simulink model "ship_template"  (R2021b)
settings: Solver=ode23t  StartTime=0.0  StopTime=60*2  MaxStep=0.1  RelTol=1e-3  AbsTol=1e-3
model workspace (MAT data in the model file):
  L = 1.2
  W = 1.2
undefined symbols (not defined in the file or in its folder): blue, blue0, blue1, blue2, centre, green, green0, green1, green2, left, Left, llx, lly, Mid, red, red0, red1, red2, right, Right, ulx, uly, X, Y, Z
libraries: sm_lib x278, nesl_utility x68, fl_lib x58, simulink x12, ee_lib x3, sdl_lib x3
(part 7 of 8)

== system ship_template/System/object scenario/9objs/contact models/object2ship/objectcontact ==
  Simscape Bus1 : SimscapeBus  HierarchyStrings=blue0;green0;red0;blue1;green1;red1;blue2;green2;red2
  Spatial Contact Force{1..6,9..11} (9 alike) : sm_lib/Forces and Torques/Spatial Contact Force  CoefficientOfDynamicFriction=0.3  CoefficientOfStaticFriction=0.5  SenseContactBaseRotation=off  SenseContactBaseTranslation=off  NormalDamping=b  NormalDampingUnits=N/(m/s)  SenseContactFollowerRotation=off  SenseContactFollowerTranslation=off  SenseContactSignal=off  NormalStiffness=k  NormalStiffnessUnits=N/m  FrictionalCriticalVelocity=1e-3  FrictionalCriticalVelocityUnits=m/s  ZeroCrossDetectContactStartAndEnd=off  FrictionType=SmoothStickSlip  SenseFrictionalForceMagnitude=off  SenseNormalForceMagnitude=off  NormalForceType=SmoothSpringDamper  SenseNormalVelocity=off  SenseSeparationDistance=off  SenseTangentialVelocity=off  SenseTangentialVelocityMagnitude=off  NormalTransitionRegionWidth=x  NormalTransitionRegionWidthUnits=m
  object : PMIOPort  Side=Left
  F : PMIOPort  Port=2  Side=Right
  connections:
  Spatial Contact Force11/RConn1 -- F/RConn1 -- Spatial Contact Force9/RConn1 -- Spatial Contact Force2/RConn1 -- Spatial Contact Force3/RConn1 -- Spatial Contact Force1/RConn1 -- Spatial Contact Force10/RConn1 -- Spatial Contact Force5/RConn1 -- Spatial Contact Force4/RConn1 -- Spatial Contact Force6/RConn1
  Spatial Contact Force10/LConn1 -- Simscape Bus1/LConn5
  Spatial Contact Force2/LConn1 -- Simscape Bus1/LConn3
  Spatial Contact Force3/LConn1 -- Simscape Bus1/LConn1
  Spatial Contact Force11/LConn1 -- Simscape Bus1/LConn6
  Spatial Contact Force1/LConn1 -- Simscape Bus1/LConn2
  Spatial Contact Force4/LConn1 -- Simscape Bus1/LConn8
  Spatial Contact Force9/LConn1 -- Simscape Bus1/LConn4
  Spatial Contact Force5/LConn1 -- Simscape Bus1/LConn9
  Spatial Contact Force6/LConn1 -- Simscape Bus1/LConn7
  Simscape Bus1/RConn1 -- object/RConn1

== system ship_template/System/object scenario/9objs/contact models/tank2collector/Subsystem ==
  Simscape Bus11 : SimscapeBus  HierarchyStrings=llx;ulx;lly;uly
  Spatial Contact Force{1,12,16..17} (4 alike) : sm_lib/Forces and Torques/Spatial Contact Force  CoefficientOfDynamicFriction=0.3  CoefficientOfStaticFriction=0.5  SenseContactBaseRotation=off  SenseContactBaseTranslation=off  NormalDamping=b  NormalDampingUnits=N/(m/s)  SenseContactFollowerRotation=off  SenseContactFollowerTranslation=off  SenseContactSignal=off  NormalStiffness=k  NormalStiffnessUnits=N/m  FrictionalCriticalVelocity=1e-3  FrictionalCriticalVelocityUnits=m/s  ZeroCrossDetectContactStartAndEnd=off  FrictionType=SmoothStickSlip  SenseFrictionalForceMagnitude=off  SenseNormalForceMagnitude=off  NormalForceType=SmoothSpringDamper  SenseNormalVelocity=off  SenseSeparationDistance=off  SenseTangentialVelocity=off  SenseTangentialVelocityMagnitude=off  NormalTransitionRegionWidth=x  NormalTransitionRegionWidthUnits=m
  tank wall : PMIOPort  Side=Left
  F : PMIOPort  Port=2  Side=Right
  connections:
  Simscape Bus11/LConn3 -- Spatial Contact Force16/LConn1
  Spatial Contact Force17/LConn1 -- Simscape Bus11/LConn1
  Spatial Contact Force16/RConn1 -- Spatial Contact Force1/RConn1 -- F/RConn1 -- Spatial Contact Force17/RConn1 -- Spatial Contact Force12/RConn1
  Simscape Bus11/LConn4 -- Spatial Contact Force1/LConn1
  tank wall/RConn1 -- Simscape Bus11/RConn1
  Simscape Bus11/LConn2 -- Spatial Contact Force12/LConn1

== system ship_template/System/object scenario/9objs/contact models/tank2collector/Subsystem1 ==
  Simscape Bus11 : SimscapeBus  HierarchyStrings=llx;ulx;lly;uly
  Spatial Contact Force{1,12,16..17} (4 alike) : sm_lib/Forces and Torques/Spatial Contact Force  CoefficientOfDynamicFriction=0.3  CoefficientOfStaticFriction=0.5  SenseContactBaseRotation=off  SenseContactBaseTranslation=off  NormalDamping=b  NormalDampingUnits=N/(m/s)  SenseContactFollowerRotation=off  SenseContactFollowerTranslation=off  SenseContactSignal=off  NormalStiffness=k  NormalStiffnessUnits=N/m  FrictionalCriticalVelocity=1e-3  FrictionalCriticalVelocityUnits=m/s  ZeroCrossDetectContactStartAndEnd=off  FrictionType=SmoothStickSlip  SenseFrictionalForceMagnitude=off  SenseNormalForceMagnitude=off  NormalForceType=SmoothSpringDamper  SenseNormalVelocity=off  SenseSeparationDistance=off  SenseTangentialVelocity=off  SenseTangentialVelocityMagnitude=off  NormalTransitionRegionWidth=x  NormalTransitionRegionWidthUnits=m
  tank wall : PMIOPort  Side=Left
  F : PMIOPort  Port=2  Side=Right
  connections:
  Simscape Bus11/LConn2 -- Spatial Contact Force12/LConn1
  tank wall/RConn1 -- Simscape Bus11/RConn1
  Simscape Bus11/LConn4 -- Spatial Contact Force1/LConn1
  F/RConn1 -- Spatial Contact Force12/RConn1 -- Spatial Contact Force17/RConn1 -- Spatial Contact Force16/RConn1 -- Spatial Contact Force1/RConn1
  Spatial Contact Force17/LConn1 -- Simscape Bus11/LConn1
  Simscape Bus11/LConn3 -- Spatial Contact Force16/LConn1

== system ship_template/System/object scenario/9objs/contact models/tank2collector/Subsystem2 ==
  Simscape Bus11 : SimscapeBus  HierarchyStrings=llx;ulx;lly;uly
  Spatial Contact Force{1,12,16..17} (4 alike) : sm_lib/Forces and Torques/Spatial Contact Force  CoefficientOfDynamicFriction=0.3  CoefficientOfStaticFriction=0.5  SenseContactBaseRotation=off  SenseContactBaseTranslation=off  NormalDamping=b  NormalDampingUnits=N/(m/s)  SenseContactFollowerRotation=off  SenseContactFollowerTranslation=off  SenseContactSignal=off  NormalStiffness=k  NormalStiffnessUnits=N/m  FrictionalCriticalVelocity=1e-3  FrictionalCriticalVelocityUnits=m/s  ZeroCrossDetectContactStartAndEnd=off  FrictionType=SmoothStickSlip  SenseFrictionalForceMagnitude=off  SenseNormalForceMagnitude=off  NormalForceType=SmoothSpringDamper  SenseNormalVelocity=off  SenseSeparationDistance=off  SenseTangentialVelocity=off  SenseTangentialVelocityMagnitude=off  NormalTransitionRegionWidth=x  NormalTransitionRegionWidthUnits=m
  tank wall : PMIOPort  Side=Left
  F : PMIOPort  Port=2  Side=Right
  connections:
  Simscape Bus11/LConn3 -- Spatial Contact Force16/LConn1
  Spatial Contact Force17/LConn1 -- Simscape Bus11/LConn1
  Spatial Contact Force1/RConn1 -- Spatial Contact Force16/RConn1 -- Spatial Contact Force17/RConn1 -- Spatial Contact Force12/RConn1 -- F/RConn1
  Simscape Bus11/LConn4 -- Spatial Contact Force1/LConn1
  tank wall/RConn1 -- Simscape Bus11/RConn1
  Simscape Bus11/LConn2 -- Spatial Contact Force12/LConn1

== system ship_template/System/object scenario/9objs/objects/object location/checkCollected ==
  xy : Inport
  Compare To Constant : simulink/Logic and Bit Operations/Compare To Constant  relop=<=  const=homeRadius  OutDataTypeStr=boolean
  Constant : Constant  Value=[Xhome, Yhome]
  Sqrt : Sqrt  SaturateOnIntegerOverflow=on
  Square : Math  Operator=square  SaturateOnIntegerOverflow=on
  Sum : Sum  Inputs=|-+
  Sum of Elements : Sum  Inputs=+
  collectFlag : Outport
  wires:
  Sum of Elements/1 -> Sqrt/1
  Sqrt/1 -> Compare To Constant/1  "dist"
  xy/1 -> Sum/1
  Square/1 -> Sum of Elements/1
  Compare To Constant/1 -> collectFlag/1  "collected"
  Constant/1 -> Sum/2
  Sum/1 -> Square/1

== system ship_template/System/object scenario/9objs/objects/object location/checkCollected1 ==
  xy : Inport
  Compare To Constant : simulink/Logic and Bit Operations/Compare To Constant  relop=<=  const=homeRadius  OutDataTypeStr=boolean
  Constant : Constant  Value=[Xhome, Yhome]
  Sqrt : Sqrt  SaturateOnIntegerOverflow=on
  Square : Math  Operator=square  SaturateOnIntegerOverflow=on
  Sum : Sum  Inputs=|-+
  Sum of Elements : Sum  Inputs=+
  collectFlag : Outport
  wires:
  Sum/1 -> Square/1
  Constant/1 -> Sum/2
  Compare To Constant/1 -> collectFlag/1  "collected"
  Square/1 -> Sum of Elements/1
  xy/1 -> Sum/1
  Sqrt/1 -> Compare To Constant/1  "dist"
  Sum of Elements/1 -> Sqrt/1

== system ship_template/System/object scenario/9objs/objects/object location/checkCollected2 ==
  xy : Inport
  Compare To Constant : simulink/Logic and Bit Operations/Compare To Constant  relop=<=  const=homeRadius  OutDataTypeStr=boolean
  Constant : Constant  Value=[Xhome, Yhome]
  Sqrt : Sqrt  SaturateOnIntegerOverflow=on
  Square : Math  Operator=square  SaturateOnIntegerOverflow=on
  Sum : Sum  Inputs=|-+
  Sum of Elements : Sum  Inputs=+
  collectFlag : Outport
  wires:
  Sum of Elements/1 -> Sqrt/1
  Sqrt/1 -> Compare To Constant/1  "dist"
  xy/1 -> Sum/1
  Square/1 -> Sum of Elements/1
  Compare To Constant/1 -> collectFlag/1  "collected"
  Constant/1 -> Sum/2
  Sum/1 -> Square/1

== system ship_template/System/object scenario/9objs/objects/object location/checkCollected3 ==
  xy : Inport
  Compare To Constant : simulink/Logic and Bit Operations/Compare To Constant  relop=<=  const=homeRadius  OutDataTypeStr=boolean
  Constant : Constant  Value=[Xhome, Yhome]
  Sqrt : Sqrt  SaturateOnIntegerOverflow=on
  Square : Math  Operator=square  SaturateOnIntegerOverflow=on
  Sum : Sum  Inputs=|-+
  Sum of Elements : Sum  Inputs=+
  collectFlag : Outport
  wires:
  Sum/1 -> Square/1
  Constant/1 -> Sum/2
  Compare To Constant/1 -> collectFlag/1  "collected"
  Square/1 -> Sum of Elements/1
  xy/1 -> Sum/1
  Sqrt/1 -> Compare To Constant/1  "dist"
  Sum of Elements/1 -> Sqrt/1

== system ship_template/System/object scenario/9objs/objects/object location/checkCollected4 ==
  xy : Inport
  Compare To Constant : simulink/Logic and Bit Operations/Compare To Constant  relop=<=  const=homeRadius  OutDataTypeStr=boolean
  Constant : Constant  Value=[Xhome, Yhome]
  Sqrt : Sqrt  SaturateOnIntegerOverflow=on
  Square : Math  Operator=square  SaturateOnIntegerOverflow=on
  Sum : Sum  Inputs=|-+
  Sum of Elements : Sum  Inputs=+
  collectFlag : Outport
  wires:
  Sum of Elements/1 -> Sqrt/1
  Sqrt/1 -> Compare To Constant/1  "dist"
  xy/1 -> Sum/1
  Square/1 -> Sum of Elements/1
  Compare To Constant/1 -> collectFlag/1  "collected"
  Constant/1 -> Sum/2
  Sum/1 -> Square/1

== system ship_template/System/object scenario/9objs/objects/object location/checkCollected5 ==
  xy : Inport
  Compare To Constant : simulink/Logic and Bit Operations/Compare To Constant  relop=<=  const=homeRadius  OutDataTypeStr=boolean
  Constant : Constant  Value=[Xhome, Yhome]
  Sqrt : Sqrt  SaturateOnIntegerOverflow=on
  Square : Math  Operator=square  SaturateOnIntegerOverflow=on
  Sum : Sum  Inputs=|-+
  Sum of Elements : Sum  Inputs=+
  collectFlag : Outport
  wires:
  Sum/1 -> Square/1
  Constant/1 -> Sum/2
  Compare To Constant/1 -> collectFlag/1  "collected"
  Square/1 -> Sum of Elements/1
  xy/1 -> Sum/1
  Sqrt/1 -> Compare To Constant/1  "dist"
  Sum of Elements/1 -> Sqrt/1

== system ship_template/System/object scenario/9objs/objects/object location/checkCollected6 ==
  xy : Inport
  Compare To Constant : simulink/Logic and Bit Operations/Compare To Constant  relop=<=  const=homeRadius  OutDataTypeStr=boolean
  Constant : Constant  Value=[Xhome, Yhome]
  Sqrt : Sqrt  SaturateOnIntegerOverflow=on
  Square : Math  Operator=square  SaturateOnIntegerOverflow=on
  Sum : Sum  Inputs=|-+
  Sum of Elements : Sum  Inputs=+
  collectFlag : Outport
  wires:
  Sum of Elements/1 -> Sqrt/1
  Sqrt/1 -> Compare To Constant/1  "dist"
  xy/1 -> Sum/1
  Square/1 -> Sum of Elements/1
  Compare To Constant/1 -> collectFlag/1  "collected"
  Constant/1 -> Sum/2
  Sum/1 -> Square/1

== system ship_template/System/object scenario/9objs/objects/object location/checkCollected7 ==
  xy : Inport
  Compare To Constant : simulink/Logic and Bit Operations/Compare To Constant  relop=<=  const=homeRadius  OutDataTypeStr=boolean
  Constant : Constant  Value=[Xhome, Yhome]
  Sqrt : Sqrt  SaturateOnIntegerOverflow=on
  Square : Math  Operator=square  SaturateOnIntegerOverflow=on
  Sum : Sum  Inputs=|-+
  Sum of Elements : Sum  Inputs=+
  collectFlag : Outport
  wires:
  Sum/1 -> Square/1
  Constant/1 -> Sum/2
  Compare To Constant/1 -> collectFlag/1  "collected"
  Square/1 -> Sum of Elements/1
  xy/1 -> Sum/1
  Sqrt/1 -> Compare To Constant/1  "dist"
  Sum of Elements/1 -> Sqrt/1

== system ship_template/System/object scenario/9objs/objects/object location/checkCollected8 ==
  xy : Inport
  Compare To Constant : simulink/Logic and Bit Operations/Compare To Constant  relop=<=  const=homeRadius  OutDataTypeStr=boolean
  Constant : Constant  Value=[Xhome, Yhome]
  Sqrt : Sqrt  SaturateOnIntegerOverflow=on
  Square : Math  Operator=square  SaturateOnIntegerOverflow=on
  Sum : Sum  Inputs=|-+
  Sum of Elements : Sum  Inputs=+
  collectFlag : Outport
  wires:
  Sum of Elements/1 -> Sqrt/1
  Sqrt/1 -> Compare To Constant/1  "dist"
  xy/1 -> Sum/1
  Square/1 -> Sum of Elements/1
  Compare To Constant/1 -> collectFlag/1  "collected"
  Constant/1 -> Sum/2
  Sum/1 -> Square/1

== system ship_template/System/object scenario/9objs/objects/object location/transform sensor ==
  Mux1 : Mux  Inputs=2
  PS-Simulink Converter : nesl_utility/PS-Simulink Converter  PhysicalDomain=network_engine_domain  SubClassName=ps_output  LeftPortType=input  RightPortType=output  PseudoPeriodic=off  Frequencies=[]  Unit=inherit  AffineConversion=off
      settings: SourceProductBaseCode=PW,SS
  PS-Simulink Converter1 : nesl_utility/PS-Simulink Converter  PhysicalDomain=network_engine_domain  SubClassName=ps_output  LeftPortType=input  RightPortType=output  PseudoPeriodic=off  Frequencies=[]  Unit=inherit  AffineConversion=off
      settings: SourceProductBaseCode=PW,SS
  Transform Sensor : sm_lib/Frames and Transforms/Transform Sensor  MeasurementFrame=World  SenseAngle=off  SenseAxis=off  SenseAngle1=off  SenseAngle2=off  SenseAngle3=off  SenseQ=off  SenseR=off  SenseOmegaX=off  SenseOmegaY=off  SenseOmegaZ=off  SenseOmega1=off  SenseOmega2=off  SenseOmega3=off  SenseQDot=off  SenseRDot=off  SenseAlphaX=off  SenseAlphaY=off  SenseAlphaZ=off  SenseAlpha1=off  SenseAlpha2=off  SenseAlpha3=off  SenseQDDot=off  SenseRDDot=off  SenseX=on  SenseY=on  SenseZ=off  SenseRad=off  SenseAzim=off  SenseDist=off  SenseInc=off  SenseXDot=off  SenseYDot=off  SenseZDot=off  SenseRadDot=off  SenseAzimDot=off  SenseDistDot=off  SenseIncDot=off  SenseXDDot=off  SenseYDDot=off  SenseZDDot=off  SenseRadDDot=off  SenseAzimDDot=off  SenseDistDDot=off  SenseIncDDot=off
  WF : PMIOPort  Side=Left
  F : PMIOPort  Port=2  Side=Right
  xy : Outport
  wires:
  PS-Simulink Converter1/1 -> Mux1/2
  Mux1/1 -> xy/1
  PS-Simulink Converter/1 -> Mux1/1
  connections:
  PS-Simulink Converter1/LConn1 -- Transform Sensor/RConn3
  PS-Simulink Converter/LConn1 -- Transform Sensor/RConn2
  WF/RConn1 -- Transform Sensor/LConn1
  Transform Sensor/RConn1 -- F/RConn1

== system ship_template/System/object scenario/9objs/objects/object location/transform sensor1 ==
  Mux1 : Mux  Inputs=2
  PS-Simulink Converter : nesl_utility/PS-Simulink Converter  PhysicalDomain=network_engine_domain  SubClassName=ps_output  LeftPortType=input  RightPortType=output  PseudoPeriodic=off  Frequencies=[]  Unit=inherit  AffineConversion=off
      settings: SourceProductBaseCode=PW,SS
  PS-Simulink Converter1 : nesl_utility/PS-Simulink Converter  PhysicalDomain=network_engine_domain  SubClassName=ps_output  LeftPortType=input  RightPortType=output  PseudoPeriodic=off  Frequencies=[]  Unit=inherit  AffineConversion=off
      settings: SourceProductBaseCode=PW,SS
  Transform Sensor : sm_lib/Frames and Transforms/Transform Sensor  MeasurementFrame=World  SenseAngle=off  SenseAxis=off  SenseAngle1=off  SenseAngle2=off  SenseAngle3=off  SenseQ=off  SenseR=off  SenseOmegaX=off  SenseOmegaY=off  SenseOmegaZ=off  SenseOmega1=off  SenseOmega2=off  SenseOmega3=off  SenseQDot=off  SenseRDot=off  SenseAlphaX=off  SenseAlphaY=off  SenseAlphaZ=off  SenseAlpha1=off  SenseAlpha2=off  SenseAlpha3=off  SenseQDDot=off  SenseRDDot=off  SenseX=on  SenseY=on  SenseZ=off  SenseRad=off  SenseAzim=off  SenseDist=off  SenseInc=off  SenseXDot=off  SenseYDot=off  SenseZDot=off  SenseRadDot=off  SenseAzimDot=off  SenseDistDot=off  SenseIncDot=off  SenseXDDot=off  SenseYDDot=off  SenseZDDot=off  SenseRadDDot=off  SenseAzimDDot=off  SenseDistDDot=off  SenseIncDDot=off
  WF : PMIOPort  Side=Left
  F : PMIOPort  Port=2  Side=Right
  xy : Outport
  wires:
  PS-Simulink Converter/1 -> Mux1/1
  Mux1/1 -> xy/1
  PS-Simulink Converter1/1 -> Mux1/2
  connections:
  Transform Sensor/RConn1 -- F/RConn1
  WF/RConn1 -- Transform Sensor/LConn1
  PS-Simulink Converter/LConn1 -- Transform Sensor/RConn2
  PS-Simulink Converter1/LConn1 -- Transform Sensor/RConn3

== system ship_template/System/object scenario/9objs/objects/object location/transform sensor2 ==
  Mux1 : Mux  Inputs=2
  PS-Simulink Converter : nesl_utility/PS-Simulink Converter  PhysicalDomain=network_engine_domain  SubClassName=ps_output  LeftPortType=input  RightPortType=output  PseudoPeriodic=off  Frequencies=[]  Unit=inherit  AffineConversion=off
      settings: SourceProductBaseCode=PW,SS
  PS-Simulink Converter1 : nesl_utility/PS-Simulink Converter  PhysicalDomain=network_engine_domain  SubClassName=ps_output  LeftPortType=input  RightPortType=output  PseudoPeriodic=off  Frequencies=[]  Unit=inherit  AffineConversion=off
      settings: SourceProductBaseCode=PW,SS
  Transform Sensor : sm_lib/Frames and Transforms/Transform Sensor  MeasurementFrame=World  SenseAngle=off  SenseAxis=off  SenseAngle1=off  SenseAngle2=off  SenseAngle3=off  SenseQ=off  SenseR=off  SenseOmegaX=off  SenseOmegaY=off  SenseOmegaZ=off  SenseOmega1=off  SenseOmega2=off  SenseOmega3=off  SenseQDot=off  SenseRDot=off  SenseAlphaX=off  SenseAlphaY=off  SenseAlphaZ=off  SenseAlpha1=off  SenseAlpha2=off  SenseAlpha3=off  SenseQDDot=off  SenseRDDot=off  SenseX=on  SenseY=on  SenseZ=off  SenseRad=off  SenseAzim=off  SenseDist=off  SenseInc=off  SenseXDot=off  SenseYDot=off  SenseZDot=off  SenseRadDot=off  SenseAzimDot=off  SenseDistDot=off  SenseIncDot=off  SenseXDDot=off  SenseYDDot=off  SenseZDDot=off  SenseRadDDot=off  SenseAzimDDot=off  SenseDistDDot=off  SenseIncDDot=off
  WF : PMIOPort  Side=Left
  F : PMIOPort  Port=2  Side=Right
  xy : Outport
  wires:
  PS-Simulink Converter1/1 -> Mux1/2
  Mux1/1 -> xy/1
  PS-Simulink Converter/1 -> Mux1/1
  connections:
  PS-Simulink Converter1/LConn1 -- Transform Sensor/RConn3
  PS-Simulink Converter/LConn1 -- Transform Sensor/RConn2
  WF/RConn1 -- Transform Sensor/LConn1
  Transform Sensor/RConn1 -- F/RConn1

== system ship_template/System/object scenario/9objs/objects/object location/transform sensor3 ==
  Mux1 : Mux  Inputs=2
  PS-Simulink Converter : nesl_utility/PS-Simulink Converter  PhysicalDomain=network_engine_domain  SubClassName=ps_output  LeftPortType=input  RightPortType=output  PseudoPeriodic=off  Frequencies=[]  Unit=inherit  AffineConversion=off
      settings: SourceProductBaseCode=PW,SS
  PS-Simulink Converter1 : nesl_utility/PS-Simulink Converter  PhysicalDomain=network_engine_domain  SubClassName=ps_output  LeftPortType=input  RightPortType=output  PseudoPeriodic=off  Frequencies=[]  Unit=inherit  AffineConversion=off
      settings: SourceProductBaseCode=PW,SS
  Transform Sensor : sm_lib/Frames and Transforms/Transform Sensor  MeasurementFrame=World  SenseAngle=off  SenseAxis=off  SenseAngle1=off  SenseAngle2=off  SenseAngle3=off  SenseQ=off  SenseR=off  SenseOmegaX=off  SenseOmegaY=off  SenseOmegaZ=off  SenseOmega1=off  SenseOmega2=off  SenseOmega3=off  SenseQDot=off  SenseRDot=off  SenseAlphaX=off  SenseAlphaY=off  SenseAlphaZ=off  SenseAlpha1=off  SenseAlpha2=off  SenseAlpha3=off  SenseQDDot=off  SenseRDDot=off  SenseX=on  SenseY=on  SenseZ=off  SenseRad=off  SenseAzim=off  SenseDist=off  SenseInc=off  SenseXDot=off  SenseYDot=off  SenseZDot=off  SenseRadDot=off  SenseAzimDot=off  SenseDistDot=off  SenseIncDot=off  SenseXDDot=off  SenseYDDot=off  SenseZDDot=off  SenseRadDDot=off  SenseAzimDDot=off  SenseDistDDot=off  SenseIncDDot=off
  WF : PMIOPort  Side=Left
  F : PMIOPort  Port=2  Side=Right
  xy : Outport
  wires:
  PS-Simulink Converter/1 -> Mux1/1
  Mux1/1 -> xy/1
  PS-Simulink Converter1/1 -> Mux1/2
  connections:
  Transform Sensor/RConn1 -- F/RConn1
  WF/RConn1 -- Transform Sensor/LConn1
  PS-Simulink Converter/LConn1 -- Transform Sensor/RConn2
  PS-Simulink Converter1/LConn1 -- Transform Sensor/RConn3

== system ship_template/System/object scenario/9objs/objects/object location/transform sensor4 ==
  Mux1 : Mux  Inputs=2
  PS-Simulink Converter : nesl_utility/PS-Simulink Converter  PhysicalDomain=network_engine_domain  SubClassName=ps_output  LeftPortType=input  RightPortType=output  PseudoPeriodic=off  Frequencies=[]  Unit=inherit  AffineConversion=off
      settings: SourceProductBaseCode=PW,SS
  PS-Simulink Converter1 : nesl_utility/PS-Simulink Converter  PhysicalDomain=network_engine_domain  SubClassName=ps_output  LeftPortType=input  RightPortType=output  PseudoPeriodic=off  Frequencies=[]  Unit=inherit  AffineConversion=off
      settings: SourceProductBaseCode=PW,SS
  Transform Sensor : sm_lib/Frames and Transforms/Transform Sensor  MeasurementFrame=World  SenseAngle=off  SenseAxis=off  SenseAngle1=off  SenseAngle2=off  SenseAngle3=off  SenseQ=off  SenseR=off  SenseOmegaX=off  SenseOmegaY=off  SenseOmegaZ=off  SenseOmega1=off  SenseOmega2=off  SenseOmega3=off  SenseQDot=off  SenseRDot=off  SenseAlphaX=off  SenseAlphaY=off  SenseAlphaZ=off  SenseAlpha1=off  SenseAlpha2=off  SenseAlpha3=off  SenseQDDot=off  SenseRDDot=off  SenseX=on  SenseY=on  SenseZ=off  SenseRad=off  SenseAzim=off  SenseDist=off  SenseInc=off  SenseXDot=off  SenseYDot=off  SenseZDot=off  SenseRadDot=off  SenseAzimDot=off  SenseDistDot=off  SenseIncDot=off  SenseXDDot=off  SenseYDDot=off  SenseZDDot=off  SenseRadDDot=off  SenseAzimDDot=off  SenseDistDDot=off  SenseIncDDot=off
  WF : PMIOPort  Side=Left
  F : PMIOPort  Port=2  Side=Right
  xy : Outport
  wires:
  PS-Simulink Converter1/1 -> Mux1/2
  Mux1/1 -> xy/1
  PS-Simulink Converter/1 -> Mux1/1
  connections:
  PS-Simulink Converter1/LConn1 -- Transform Sensor/RConn3
  PS-Simulink Converter/LConn1 -- Transform Sensor/RConn2
  WF/RConn1 -- Transform Sensor/LConn1
  Transform Sensor/RConn1 -- F/RConn1

== system ship_template/System/object scenario/9objs/objects/object location/transform sensor5 ==
  Mux1 : Mux  Inputs=2
  PS-Simulink Converter : nesl_utility/PS-Simulink Converter  PhysicalDomain=network_engine_domain  SubClassName=ps_output  LeftPortType=input  RightPortType=output  PseudoPeriodic=off  Frequencies=[]  Unit=inherit  AffineConversion=off
      settings: SourceProductBaseCode=PW,SS
  PS-Simulink Converter1 : nesl_utility/PS-Simulink Converter  PhysicalDomain=network_engine_domain  SubClassName=ps_output  LeftPortType=input  RightPortType=output  PseudoPeriodic=off  Frequencies=[]  Unit=inherit  AffineConversion=off
      settings: SourceProductBaseCode=PW,SS
  Transform Sensor : sm_lib/Frames and Transforms/Transform Sensor  MeasurementFrame=World  SenseAngle=off  SenseAxis=off  SenseAngle1=off  SenseAngle2=off  SenseAngle3=off  SenseQ=off  SenseR=off  SenseOmegaX=off  SenseOmegaY=off  SenseOmegaZ=off  SenseOmega1=off  SenseOmega2=off  SenseOmega3=off  SenseQDot=off  SenseRDot=off  SenseAlphaX=off  SenseAlphaY=off  SenseAlphaZ=off  SenseAlpha1=off  SenseAlpha2=off  SenseAlpha3=off  SenseQDDot=off  SenseRDDot=off  SenseX=on  SenseY=on  SenseZ=off  SenseRad=off  SenseAzim=off  SenseDist=off  SenseInc=off  SenseXDot=off  SenseYDot=off  SenseZDot=off  SenseRadDot=off  SenseAzimDot=off  SenseDistDot=off  SenseIncDot=off  SenseXDDot=off  SenseYDDot=off  SenseZDDot=off  SenseRadDDot=off  SenseAzimDDot=off  SenseDistDDot=off  SenseIncDDot=off
  WF : PMIOPort  Side=Left
  F : PMIOPort  Port=2  Side=Right
  xy : Outport
  wires:
  PS-Simulink Converter/1 -> Mux1/1
  Mux1/1 -> xy/1
  PS-Simulink Converter1/1 -> Mux1/2
  connections:
  Transform Sensor/RConn1 -- F/RConn1
  WF/RConn1 -- Transform Sensor/LConn1
  PS-Simulink Converter/LConn1 -- Transform Sensor/RConn2
  PS-Simulink Converter1/LConn1 -- Transform Sensor/RConn3

== system ship_template/System/object scenario/9objs/objects/object location/transform sensor6 ==
  Mux1 : Mux  Inputs=2
  PS-Simulink Converter : nesl_utility/PS-Simulink Converter  PhysicalDomain=network_engine_domain  SubClassName=ps_output  LeftPortType=input  RightPortType=output  PseudoPeriodic=off  Frequencies=[]  Unit=inherit  AffineConversion=off
      settings: SourceProductBaseCode=PW,SS
  PS-Simulink Converter1 : nesl_utility/PS-Simulink Converter  PhysicalDomain=network_engine_domain  SubClassName=ps_output  LeftPortType=input  RightPortType=output  PseudoPeriodic=off  Frequencies=[]  Unit=inherit  AffineConversion=off
      settings: SourceProductBaseCode=PW,SS
  Transform Sensor : sm_lib/Frames and Transforms/Transform Sensor  MeasurementFrame=World  SenseAngle=off  SenseAxis=off  SenseAngle1=off  SenseAngle2=off  SenseAngle3=off  SenseQ=off  SenseR=off  SenseOmegaX=off  SenseOmegaY=off  SenseOmegaZ=off  SenseOmega1=off  SenseOmega2=off  SenseOmega3=off  SenseQDot=off  SenseRDot=off  SenseAlphaX=off  SenseAlphaY=off  SenseAlphaZ=off  SenseAlpha1=off  SenseAlpha2=off  SenseAlpha3=off  SenseQDDot=off  SenseRDDot=off  SenseX=on  SenseY=on  SenseZ=off  SenseRad=off  SenseAzim=off  SenseDist=off  SenseInc=off  SenseXDot=off  SenseYDot=off  SenseZDot=off  SenseRadDot=off  SenseAzimDot=off  SenseDistDot=off  SenseIncDot=off  SenseXDDot=off  SenseYDDot=off  SenseZDDot=off  SenseRadDDot=off  SenseAzimDDot=off  SenseDistDDot=off  SenseIncDDot=off
  WF : PMIOPort  Side=Left
  F : PMIOPort  Port=2  Side=Right
  xy : Outport
  wires:
  PS-Simulink Converter1/1 -> Mux1/2
  Mux1/1 -> xy/1
  PS-Simulink Converter/1 -> Mux1/1
  connections:
  PS-Simulink Converter1/LConn1 -- Transform Sensor/RConn3
  PS-Simulink Converter/LConn1 -- Transform Sensor/RConn2
  WF/RConn1 -- Transform Sensor/LConn1
  Transform Sensor/RConn1 -- F/RConn1

== system ship_template/System/object scenario/9objs/objects/object location/transform sensor7 ==
  Mux1 : Mux  Inputs=2
  PS-Simulink Converter : nesl_utility/PS-Simulink Converter  PhysicalDomain=network_engine_domain  SubClassName=ps_output  LeftPortType=input  RightPortType=output  PseudoPeriodic=off  Frequencies=[]  Unit=inherit  AffineConversion=off
      settings: SourceProductBaseCode=PW,SS
  PS-Simulink Converter1 : nesl_utility/PS-Simulink Converter  PhysicalDomain=network_engine_domain  SubClassName=ps_output  LeftPortType=input  RightPortType=output  PseudoPeriodic=off  Frequencies=[]  Unit=inherit  AffineConversion=off
      settings: SourceProductBaseCode=PW,SS
  Transform Sensor : sm_lib/Frames and Transforms/Transform Sensor  MeasurementFrame=World  SenseAngle=off  SenseAxis=off  SenseAngle1=off  SenseAngle2=off  SenseAngle3=off  SenseQ=off  SenseR=off  SenseOmegaX=off  SenseOmegaY=off  SenseOmegaZ=off  SenseOmega1=off  SenseOmega2=off  SenseOmega3=off  SenseQDot=off  SenseRDot=off  SenseAlphaX=off  SenseAlphaY=off  SenseAlphaZ=off  SenseAlpha1=off  SenseAlpha2=off  SenseAlpha3=off  SenseQDDot=off  SenseRDDot=off  SenseX=on  SenseY=on  SenseZ=off  SenseRad=off  SenseAzim=off  SenseDist=off  SenseInc=off  SenseXDot=off  SenseYDot=off  SenseZDot=off  SenseRadDot=off  SenseAzimDot=off  SenseDistDot=off  SenseIncDot=off  SenseXDDot=off  SenseYDDot=off  SenseZDDot=off  SenseRadDDot=off  SenseAzimDDot=off  SenseDistDDot=off  SenseIncDDot=off
  WF : PMIOPort  Side=Left
  F : PMIOPort  Port=2  Side=Right
  xy : Outport
  wires:
  PS-Simulink Converter/1 -> Mux1/1
  Mux1/1 -> xy/1
  PS-Simulink Converter1/1 -> Mux1/2
  connections:
  Transform Sensor/RConn1 -- F/RConn1
  WF/RConn1 -- Transform Sensor/LConn1
  PS-Simulink Converter/LConn1 -- Transform Sensor/RConn2
  PS-Simulink Converter1/LConn1 -- Transform Sensor/RConn3

== system ship_template/System/object scenario/9objs/objects/object location/transform sensor8 ==
  Mux1 : Mux  Inputs=2
  PS-Simulink Converter : nesl_utility/PS-Simulink Converter  PhysicalDomain=network_engine_domain  SubClassName=ps_output  LeftPortType=input  RightPortType=output  PseudoPeriodic=off  Frequencies=[]  Unit=inherit  AffineConversion=off
      settings: SourceProductBaseCode=PW,SS
  PS-Simulink Converter1 : nesl_utility/PS-Simulink Converter  PhysicalDomain=network_engine_domain  SubClassName=ps_output  LeftPortType=input  RightPortType=output  PseudoPeriodic=off  Frequencies=[]  Unit=inherit  AffineConversion=off
      settings: SourceProductBaseCode=PW,SS
  Transform Sensor : sm_lib/Frames and Transforms/Transform Sensor  MeasurementFrame=World  SenseAngle=off  SenseAxis=off  SenseAngle1=off  SenseAngle2=off  SenseAngle3=off  SenseQ=off  SenseR=off  SenseOmegaX=off  SenseOmegaY=off  SenseOmegaZ=off  SenseOmega1=off  SenseOmega2=off  SenseOmega3=off  SenseQDot=off  SenseRDot=off  SenseAlphaX=off  SenseAlphaY=off  SenseAlphaZ=off  SenseAlpha1=off  SenseAlpha2=off  SenseAlpha3=off  SenseQDDot=off  SenseRDDot=off  SenseX=on  SenseY=on  SenseZ=off  SenseRad=off  SenseAzim=off  SenseDist=off  SenseInc=off  SenseXDot=off  SenseYDot=off  SenseZDot=off  SenseRadDot=off  SenseAzimDot=off  SenseDistDot=off  SenseIncDot=off  SenseXDDot=off  SenseYDDot=off  SenseZDDot=off  SenseRadDDot=off  SenseAzimDDot=off  SenseDistDDot=off  SenseIncDDot=off
  WF : PMIOPort  Side=Left
  F : PMIOPort  Port=2  Side=Right
  xy : Outport
  wires:
  PS-Simulink Converter1/1 -> Mux1/2
  Mux1/1 -> xy/1
  PS-Simulink Converter/1 -> Mux1/1
  connections:
  PS-Simulink Converter1/LConn1 -- Transform Sensor/RConn3
  PS-Simulink Converter/LConn1 -- Transform Sensor/RConn2
  WF/RConn1 -- Transform Sensor/LConn1
  Transform Sensor/RConn1 -- F/RConn1

== system ship_template/System/propulsion and steering/one propeller and rudder (experimental)/Servo Rudder Mechanism/Drag/Subsystem ==
  PS Add : fl_lib/Physical Signals/Functions/PS Add
  PS Product1 : fl_lib/Physical Signals/Functions/PS Product
  PS Product2 : fl_lib/Physical Signals/Functions/PS Product
  cos : fl_lib/Physical Signals/Functions/PS Math Function  fcn_choice=foundation.enum.math_function.cos  v=1
      settings: SourceProductBaseCode=SS
  sin : fl_lib/Physical Signals/Functions/PS Math Function  fcn_choice=foundation.enum.math_function.sin  v=1
      settings: SourceProductBaseCode=SS
  theta : PMIOPort  Side=Left
  v_into_rudder : PMIOPort  Port=2  Side=Right
  vx : PMIOPort  Port=3  Side=Left
  vy : PMIOPort  Port=4  Side=Left
  connections:
  PS Add/LConn1 -- PS Product1/RConn1
  vx/RConn1 -- PS Product1/LConn2
  PS Product1/LConn1 -- cos/RConn1
  PS Product2/LConn1 -- sin/RConn1
  PS Product2/RConn1 -- PS Add/LConn2
  vy/RConn1 -- PS Product2/LConn2
  cos/LConn1 -- theta/RConn1 -- sin/LConn1
  PS Add/RConn1 -- v_into_rudder/RConn1

== system ship_template/System/propulsion and steering/one propeller and rudder (experimental)/Ship Locations/Motor/DC_Motor ==
  Inertia : sm_lib/Body Elements/Inertia  InertiaType=Custom  Mass=0.02322884657409609  MassUnits=kg  CenterOfMass=[0, 0, 0]  CenterOfMassUnits=m  MomentsOfInertia=[0, 1e-06, 1e-06]  MomentsOfInertiaUnits=kg*m^2  ProductsOfInertia=[0, 0, 0]  ProductsOfInertiaUnits=kg*m^2  GraphicType=None  MarkerShape=Inertia  MarkerSize=20  GraphicVisPropType=SimpleVisualProperties  GraphicDiffuseColor=[0.5 0.5 0.5]  GraphicSpecularColor=[0.5 0.5 0.5 1.0]  GraphicAmbientColor=[0.15 0.15 0.15 1.0]  GraphicEmissiveColor=[0.0 0.0 0.0 1.0]  GraphicShininess=75  GraphicOpacity=1.0
  InertiaOriginTransform : sm_lib/Frames and Transforms/Rigid Transform  TranslationMethod=Cartesian  TranslationStandardOffset=0  TranslationLengthUnit=m  TranslationStandardAxis=+Z  TranslationCartesianOffset=[-0.008861257097837374, 0.03000026436953541, -0.01000089661835722]  TranslationROffset=0  TranslationROffsetUnits=m  TranslationZOffset=0  TranslationZOffsetUnits=m  TranslationThetaOffset=0  TranslationThetaOffsetUnits=deg  RotationMethod=RotationSequence  RotationAngleUnits=deg  RotationStandardAxis=+Z  RotationAngle=0.0  RotationArbitraryAxis=[0 0 1]  FollAlignAxisA=+X  BaseAlignAxisA=+Y  FollAlignAxisB=+Y  BaseAlignAxisB=+Z  RotationSequenceAxes=BaseAxes  RotationSequence=XYZ  RotationSequenceAngles=[0, 0, 0]  RotationSequenceAnglesUnits=rad  RotationMatrix=[1 0 0; 0 1 0; 0 0 1]
  ReferenceFrame : sm_lib/Frames and Transforms/Reference Frame
  Rev2_AxisTransform : sm_lib/Frames and Transforms/Rigid Transform  TranslationMethod=Cartesian  TranslationStandardOffset=0  TranslationLengthUnit=m  TranslationStandardAxis=+Z  TranslationCartesianOffset=[0, 0, 0]  TranslationROffset=0  TranslationROffsetUnits=m  TranslationZOffset=0  TranslationZOffsetUnits=m  TranslationThetaOffset=0  TranslationThetaOffsetUnits=deg  RotationMethod=ArbitraryAxis  RotationAngleUnits=rad  RotationStandardAxis=+Z  RotationAngle=1.570796326794897  RotationArbitraryAxis=[-0, 1, 0]  FollAlignAxisA=+X  BaseAlignAxisA=+Y  FollAlignAxisB=+Y  BaseAlignAxisB=+Z  RotationSequenceAxes=FollowerAxes  RotationSequence=XYX  RotationSequenceAngles=[0 0 0]  RotationSequenceAnglesUnits=deg  RotationMatrix=[1 0 0; 0 1 0; 0 0 1]
  Rev2_OriginTransform : sm_lib/Frames and Transforms/Rigid Transform  TranslationMethod=Cartesian  TranslationStandardOffset=0  TranslationLengthUnit=m  TranslationStandardAxis=+Z  TranslationCartesianOffset=[0.0028, 0.03, -0.01]  TranslationROffset=0  TranslationROffsetUnits=m  TranslationZOffset=0  TranslationZOffsetUnits=m  TranslationThetaOffset=0  TranslationThetaOffsetUnits=deg  RotationMethod=RotationSequence  RotationAngleUnits=deg  RotationStandardAxis=+Z  RotationAngle=0.0  RotationArbitraryAxis=[0 0 1]  FollAlignAxisA=+X  BaseAlignAxisA=+Y  FollAlignAxisB=+Y  BaseAlignAxisB=+Z  RotationSequenceAxes=BaseAxes  RotationSequence=XYZ  RotationSequenceAngles=[0, 0, 0]  RotationSequenceAnglesUnits=rad  RotationMatrix=[1 0 0; 0 1 0; 0 0 1]
  Visual : sm_lib/Body Elements/File Solid  ExtGeomFileName=6331K86_Compact_Round-Face_DC_Motor_2.stl  UnitType=Custom  ExtGeomFileUnits=mm  StepReaderType=HEX  ExportConvexHullGeometry=off  InertiaType=Custom  Mass=0  MassUnits=kg  CenterOfMass=[0, 0, 0]  CenterOfMassUnits=m  MomentsOfInertia=[0, 0, 0]  MomentsOfInertiaUnits=kg*m^2  ProductsOfInertia=[0, 0, 0]  ProductsOfInertiaUnits=kg*m^2  BasedOnType=DensityFromFile  Density=1000  DensityUnits=kg/m^3  DoExposeReferenceFrame=on  SerializedFrames=<Frames/>  GraphicType=FromGeometry  MarkerShape=Sphere  MarkerSize=10  GraphicVisPropType=SimpleVisualProperties  GraphicDiffuseColor="[0.8784    0.8745    0.8588]"  GraphicSpecularColor=[0.5 0.5 0.5 1.0]  GraphicAmbientColor=[0.15 0.15 0.15 1.0]  GraphicEmissiveColor=[0.0 0.0 0.0 1.0]  GraphicShininess=75  GraphicOpacity=1
  VisualOriginTransform : sm_lib/Frames and Transforms/Rigid Transform  TranslationMethod=Cartesian  TranslationStandardOffset=0  TranslationLengthUnit=m  TranslationStandardAxis=+Z  TranslationCartesianOffset=[0.076728, -0.02883, -0.041672]  TranslationROffset=0  TranslationROffsetUnits=m  TranslationZOffset=0  TranslationZOffsetUnits=m  TranslationThetaOffset=0  TranslationThetaOffsetUnits=deg  RotationMethod=RotationSequence  RotationAngleUnits=deg  RotationStandardAxis=+Z  RotationAngle=0.0  RotationArbitraryAxis=[0 0 1]  FollAlignAxisA=+X  BaseAlignAxisA=+Y  FollAlignAxisB=+Y  BaseAlignAxisB=+Z  RotationSequenceAxes=BaseAxes  RotationSequence=XYZ  RotationSequenceAngles=[0, 0, 0]  RotationSequenceAnglesUnits=rad  RotationMatrix=[1 0 0; 0 1 0; 0 0 1]
  F : PMIOPort  Side=Left
  F1 : PMIOPort  Port=2  Side=Right
  connections:
  Visual/RConn1 -- VisualOriginTransform/RConn1
  Rev2_AxisTransform/LConn1 -- Rev2_OriginTransform/RConn1
  Rev2_AxisTransform/RConn1 -- F1/RConn1
  F/RConn1 -- VisualOriginTransform/LConn1 -- Rev2_OriginTransform/LConn1 -- InertiaOriginTransform/LConn1 -- ReferenceFrame/RConn1
  Inertia/RConn1 -- InertiaOriginTransform/RConn1

== system ship_template/System/propulsion and steering/one propeller and rudder (experimental)/Ship Locations/Motor/Mixer_Propeller_2 ==
  ReferenceFrame : sm_lib/Frames and Transforms/Reference Frame
  Rev2_AxisInvTransform : sm_lib/Frames and Transforms/Rigid Transform  TranslationMethod=Cartesian  TranslationStandardOffset=0  TranslationLengthUnit=m  TranslationStandardAxis=+Z  TranslationCartesianOffset=[0, 0, 0]  TranslationROffset=0  TranslationROffsetUnits=m  TranslationZOffset=0  TranslationZOffsetUnits=m  TranslationThetaOffset=0  TranslationThetaOffsetUnits=deg  RotationMethod=ArbitraryAxis  RotationAngleUnits=rad  RotationStandardAxis=+Z  RotationAngle=1.570796326794897  RotationArbitraryAxis=[-0, 1, 0]  FollAlignAxisA=+X  BaseAlignAxisA=+Y  FollAlignAxisB=+Y  BaseAlignAxisB=+Z  RotationSequenceAxes=FollowerAxes  RotationSequence=XYX  RotationSequenceAngles=[0 0 0]  RotationSequenceAnglesUnits=deg  RotationMatrix=[1 0 0; 0 1 0; 0 0 1]
  Visual : sm_lib/Body Elements/File Solid  ExtGeomFileName=8004K13_Stainless_Steel_Mixer_Propeller_2.stl  UnitType=Custom  ExtGeomFileUnits=mm  StepReaderType=HEX  ExportConvexHullGeometry=off  InertiaType=Custom  Mass=0  MassUnits=kg  CenterOfMass=[0, 0, 0]  CenterOfMassUnits=m  MomentsOfInertia=[0, 0, 0]  MomentsOfInertiaUnits=kg*m^2  ProductsOfInertia=[0, 0, 0]  ProductsOfInertiaUnits=kg*m^2  BasedOnType=DensityFromFile  Density=1000  DensityUnits=kg/m^3  DoExposeReferenceFrame=on  SerializedFrames=<Frames/>  GraphicType=FromGeometry  MarkerShape=Sphere  MarkerSize=10  GraphicVisPropType=SimpleVisualProperties  GraphicDiffuseColor=[0.0 0.8 0.2]  GraphicSpecularColor=[0.5 0.5 0.5 1.0]  GraphicAmbientColor=[0.15 0.15 0.15 1.0]  GraphicEmissiveColor=[0.0 0.0 0.0 1.0]  GraphicShininess=75  GraphicOpacity=1
  VisualOriginTransform : sm_lib/Frames and Transforms/Rigid Transform  TranslationMethod=Cartesian  TranslationStandardOffset=0  TranslationLengthUnit=m  TranslationStandardAxis=+Z  TranslationCartesianOffset=[0.07392799999999999, -0.05883, -0.031672]  TranslationROffset=0  TranslationROffsetUnits=m  TranslationZOffset=0  TranslationZOffsetUnits=m  TranslationThetaOffset=0  TranslationThetaOffsetUnits=deg  RotationMethod=RotationSequence  RotationAngleUnits=deg  RotationStandardAxis=+Z  RotationAngle=0.0  RotationArbitraryAxis=[0 0 1]  FollAlignAxisA=+X  BaseAlignAxisA=+Y  FollAlignAxisB=+Y  BaseAlignAxisB=+Z  RotationSequenceAxes=BaseAxes  RotationSequence=XYZ  RotationSequenceAngles=[0, 0, 0]  RotationSequenceAnglesUnits=rad  RotationMatrix=[1 0 0; 0 1 0; 0 0 1]
  F : PMIOPort  Side=Left
  connections:
  Visual/RConn1 -- VisualOriginTransform/RConn1
  Rev2_AxisInvTransform/RConn1 -- F/RConn1
  VisualOriginTransform/LConn1 -- Rev2_AxisInvTransform/LConn1 -- ReferenceFrame/RConn1

== system ship_template/System/propulsion and steering/one propeller and rudder (experimental)/Ship Locations/Motor/animate spin ==
  Abs : Abs
  Gain1 : Gain  Gain=1e5
  Integrator1 : Integrator
  PS-Simulink Converter2 : nesl_utility/PS-Simulink Converter  PhysicalDomain=network_engine_domain  SubClassName=ps_output  LeftPortType=input  RightPortType=output  PseudoPeriodic=off  Frequencies=[]  Unit=inherit  AffineConversion=off
      settings: SourceProductBaseCode=PW,SS
  Product : Product
  Selector : Selector  InputPortWidth=3  IndexOptions=Index vector (dialog)  Indices=1  OutputSizes=1
  Sign : Signum
  Simulink-PS Converter1 : nesl_utility/Simulink-PS Converter  PhysicalDomain=network_engine_domain  SubClassName=ps_input  LeftPortType=input  RightPortType=output  PseudoPeriodic=off  Frequencies=[]  NoiseDistribution=none  NoiseParameters=[]  Unit=1  AffineConversion=off  FilteringAndDerivatives=filter  SimscapeFilterOrder=2  InputFilterTimeConstant=0.001  UdotUserProvided=0
      settings: SourceProductBaseCode=PW,SS
  Sqrt : Sqrt  SaturateOnIntegerOverflow=on
  ft : PMIOPort  Side=Left
  q : PMIOPort  Port=2  Side=Right
  wires:
  Sign/1 -> Product/1
  Sqrt/1 -> Gain1/1
  Abs/1 -> Sqrt/1
  Product/1 -> Integrator1/1
  PS-Simulink Converter2/1 -> Selector/1
  Integrator1/1 -> Simulink-PS Converter1/1
  Selector/1 -> Abs/1, Sign/1
  Gain1/1 -> Product/2
  connections:
  Simulink-PS Converter1/RConn1 -- q/RConn1
  ft/RConn1 -- PS-Simulink Converter2/LConn1

== system ship_template/System/propulsion and steering/one propeller and rudder (experimental)/propeller thrust model/physical model/DC motor left ==
  PWM : Inport
  Controlled Voltage Source : fl_lib/Electrical/Electrical Sources/Controlled Voltage Source
  DC Motor : ee_lib/Electromechanical/Brushed Motors/DC Motor  field_option=ee.enum.field_option.pm  Rf=100 Ohm  Lf=1 H  Laf=0.15 H  If0=0 A  parameterization=ee.enum.dcparam_option.torque_speed  Ra=3.9 Ohm  La=12e-6 H  emf_or_torque=ee.enum.emf_or_torque.kv  Kv=0.072e-3 V/rpm  Ki=6.876e-4 N*m/A  T_stall=0.068 N*m  w_max=15000 rpm  w_rated=15000 rpm  P_rated=0.08 W  V_rated=6 V  lam_param=ee.enum.lam_param.damping  i_noload=0 A  V_i_noload=1.5 V  J=0.01 g*cm^2  lam=0 N*m/(rad/s)  speed0=0 rpm  enable_fault_armature=simscape.enum.onoff.off  rev_faulted=1 / 3  G_faulted_armature=1e-5 S  fault_trigger_armature=ee.enum.faults.faultTrigger.temporal  t_fault_armature=1 s  max_permissible_current_armature=inf A  t_fail_on_current_armature=1 s  enable_fault_field=simscape.enum.onoff.off  G_faulted_field=1e-5 S  fault_trigger_field=ee.enum.faults.faultTrigger.temporal  t_fault_field=1 s  max_permissible_current_field=inf A  t_fail_on_current_field=1 s  fault_action=simscape.enum.assert.action.none  alpha=3.93e-3 1/K  Tmeas=25 degC  thermal_mass=100 J/K  initial_temperature=25 degC
  Electrical Reference : fl_lib/Electrical/Electrical Elements/Electrical Reference
  Mechanical Rotational Reference : fl_lib/Mechanical/Rotational Elements/Mechanical Rotational Reference
  Simulink-PS Converter : nesl_utility/Simulink-PS Converter  PhysicalDomain=network_engine_domain  SubClassName=ps_input  LeftPortType=input  RightPortType=output  PseudoPeriodic=off  Frequencies=[]  NoiseDistribution=none  NoiseParameters=[]  Unit=1  AffineConversion=off  FilteringAndDerivatives=provide  SimscapeFilterOrder=1  InputFilterTimeConstant=0.001  UdotUserProvided=0
      settings: SourceProductBaseCode=PW,SS
  Solver Configuration : nesl_utility/Solver Configuration  PhysicalDomain=network_engine_domain  SubClassName=solver  LeftPortType=input  RightPortType=generic  Tones=[]  Harmonics=[]  SimulateNoise=off  Profile=off  UseLocalSampling=off  EnableSwitchedLinearOptims=on  FrequencyDomain=off  UseCCode=off  RelTol=0.001  AbsTol=1e-06  MinStep=1e-09  ToWorkspace=off  RevertToSquareIcSolve=off  NumHomotopyIterations=100  PhasorMode=off  PhasorModeNumHarmonics=1  DoDC=off  ResidualTolerance=1e-09  UseLocalSolver=off  LocalSolverChoice=NE_BACKWARD_EULER_ADVANCER  LocalSolverSampleTime=0.001  DoFixedCost=off  MaxNonlinIter=3  MaxModeIter=2  ComputeImpulses=off  ImpulseIterations=2  LinearAlgebra=auto  EquationFormulation=NE_TIME_EF  DelaysMemoryBudget=1024  AutomaticFiltering=on  FilteringTimeConstant=0.001  PartitionStorageMethod=AS_NEEDED  PartitionMemoryBudget=1024  PartitionMethod=ROBUST
      settings: SourceProductBaseCode=PW,SS
  V : Gain  Gain=6
  reducing gearbox : fl_lib/Mechanical/Mechanisms/Gear Box  ratio=1/150  t_in_specify=off  t_in_priority=None  t_in=0 N*m  t_in_nominal_specify=off  t_in_nominal_unit=N*m  t_in_nominal_value=1  t_out_specify=off  t_out_priority=None  t_out=0 N*m  t_out_nominal_specify=off  t_out_nominal_unit=N*m  t_out_nominal_value=1
  shaft : PMIOPort  Side=Right
  housing : PMIOPort  Port=2  Side=Right
  wires:
  PWM/1 -> V/1
  V/1 -> Simulink-PS Converter/1
  connections:
  Simulink-PS Converter/RConn1 -- Controlled Voltage Source/RConn1
  DC Motor/LConn1 -- Solver Configuration/RConn1 -- Controlled Voltage Source/LConn1
  reducing gearbox/LConn1 -- DC Motor/LConn2
  Mechanical Rotational Reference/LConn1 -- housing/RConn1 -- DC Motor/RConn2
  Controlled Voltage Source/RConn2 -- Electrical Reference/LConn1 -- DC Motor/RConn1
  reducing gearbox/RConn1 -- shaft/RConn1

== system ship_template/System/propulsion and steering/one propeller and rudder (experimental)/propeller thrust model/physical model/Propeller left ==
  Ideal Force Sensor : fl_lib/Mechanical/Mechanical Sensors/Ideal Force Sensor
  Mass1 : fl_lib/Mechanical/Translational Elements/Mass  mass=0.1 kg  num_ports=foundation.enum.numPorts2.one  v_specify=off  v_priority=High  v=0 m/s  v_nominal_specify=off  v_nominal_unit=m/s  v_nominal_value=1  f_specify=off  f_priority=None  f=0 N  f_nominal_specify=off  f_nominal_unit=N  f_nominal_value=1
  Mechanical Translational Reference : fl_lib/Mechanical/Translational Elements/Mechanical Translational Reference
  PS-Simulink Converter : nesl_utility/PS-Simulink Converter  PhysicalDomain=network_engine_domain  SubClassName=ps_output  LeftPortType=input  RightPortType=output  PseudoPeriodic=off  Frequencies=[]  Unit=inherit  AffineConversion=off
      settings: SourceProductBaseCode=PW,SS
  Propeller : sdl_lib/Engines & Motors/Propeller  parameterization=sdl.enum.PropellerParameterization.Constant  pitch_type=foundation.enum.constant_controlled.constant  D=100 mm  kt_const=0.25  kq_const=0.05  kt_poly_fixed=[.063, -.19, -.25, .37]  kq_poly_fixed=[.0043, -.021, -.03, .05]  pitch_ratio_TLU=[-.5, .5, .7, .9, 1.1, 1.4]  kt_poly_TLU=[.04, -.1, -.24, .12; .118, -.24, -.24, .19; .082, -.21, -.25, .28; .063, -.19, -.25, .37; .055, -.17, -.25, .45; .064, -.21, -.19, .55]  kq_poly_TLU=[.02, -.06, -.02, .02; .04, -.034, -.016, .018; .0076, -.02, -.023, .031; .0043, -.021, -.03, .05; .0047, -.024, -.036, .073; .0045, -.025, -.044, .11]  J_tab_TLU=[0, .3, .5, .7, .9, 1.2, 1.5]  kt_tab_fixed=[.37, .28, .21, .12, .033, -.098, -.23]  kq_tab_fixed=[.049, .039, .03, .02, .0096, -.0093, -.028]  kt_tab_TLU=[.12, .04, -.02, -.083, -.15, -.24, -.33; .19, .1, .029, -.047, -.12, -.23, -.35; .28, .19, .12, .032, -.054, -.18, -.31; .37, .28, .21, .12, .033, -.098, -.23; .45, .36, .29, .21, .13, -.0057, -.16; .54, .47, .41, .33, .25, .13, .0029]  kq_tab_TLU=[.02, .0091, -.0025, -.017, -.032, -.056, -.078; .017, .011, .006, .0009, -.0041, -.012, -.019; .03, .022, .015, .0074, -.0008, -.013, -.026; .049, .039, .03, .02, .0096, -.0093, -.028; .072, .06, .05, .038, .025, .0042, -.015; .11, .097, .085, .071, .057, .033, .0065]  interp_method=simscape.enum.interpolation.linear  extrap_method=simscape.enum.extrapolation.linear  density_spec=foundation.enum.constant_variable.constant  rho=1 kg/m^3  translational_ports=sdl.enum.ConnectionType.Conserving  wake_fraction=0.2  efficiency_sensor=simscape.enum.onoff.off  n_thr=0.001 Hz  k_thr=0.001  operation_check=simscape.enum.assert.action.warn  w_specify=off  w_priority=None  w=0 rad/s  w_nominal_specify=off  w_nominal_unit=rad/s  w_nominal_value=1  Q_specify=off  Q_priority=None  Q=0 N*m  Q_nominal_specify=off  Q_nominal_unit=N*m  Q_nominal_value=1  v_specify=off  v_priority=None  v=0 m/s  v_nominal_specify=off  v_nominal_unit=m/s  v_nominal_value=1  thrust_specify=off  thrust_priority=None  thrust=0 N  thrust_nominal_specify=off  thrust_nominal_unit=N  thrust_nominal_value=1
      settings: SourceProductBaseCode=LD  InternalSimscapePortConfiguration="{\"Bottom\":[],\"Left\":[{\"id\":\"R1\",\"label\":\"R1\",\"type\":\"foundation.mechanical.rotational.rotational\"},{\"id\":\"C1\",\"label\":\"C1\",\"type\":\"foundation.mechanical.rotational.rotational\"}],\"Right\":[{\"id\":\"R2\",\"label\":\"R2\",\"type\":\"foundation.mechanical.translational.translational\"},{\"id\":\"C2\",\"label\":\"C2\",\"type\":\"foundation.mechanical.translational.translational\"}],\"Top\":[]}"
  speed increasing : fl_lib/Mechanical/Mechanisms/Gear Box  ratio=1  t_in_specify=off  t_in_priority=None  t_in=0 N*m  t_in_nominal_specify=off  t_in_nominal_unit=N*m  t_in_nominal_value=1  t_out_specify=off  t_out_priority=None  t_out=0 N*m  t_out_nominal_specify=off  t_out_nominal_unit=N*m  t_out_nominal_value=1
  shaft : PMIOPort  Side=Left
  housing : PMIOPort  Port=2  Side=Left
  T : Outport
  wires:
  PS-Simulink Converter/1 -> T/1
  connections:
  Propeller/LConn2 -- housing/RConn1
  Ideal Force Sensor/RConn2 -- PS-Simulink Converter/LConn1
  Mass1/LConn1 -- Ideal Force Sensor/RConn1
  Propeller/RConn2 -- Mechanical Translational Reference/LConn1
  Propeller/RConn1 -- Ideal Force Sensor/LConn1
  Propeller/LConn1 -- speed increasing/RConn1
  speed increasing/LConn1 -- shaft/RConn1

== system ship_template/System/propulsion and steering/one propeller and rudder (experimental)/propeller thrust model/simulink model/motor1 ==
  PWM : Inport
  1/J : Gain  Gain=1/J
  1/R : Gain  Gain=1/R
  Gain : Gain  Gain=Vmax
  Gain3 : Gain  Gain=km
  Integrator : Integrator
  Saturation : Saturate  UpperLimit=1  LowerLimit=-1
  Sum : Sum  Inputs=|+-
  km : Gain  Gain=km
  Ω : Outport
  wires:
  Saturation/1 -> Gain/1
  Gain/1 -> Sum/1
  PWM/1 -> Saturation/1
  1/R/1 -> Gain3/1  "I"
  km/1 -> Sum/2
  Gain3/1 -> 1/J/1
  Integrator/1 -> km/1, Ω/1  "Ω"
  Sum/1 -> 1/R/1  "IR"
  1/J/1 -> Integrator/1  "dΩ/dt"

== system ship_template/System/propulsion and steering/one propeller and rudder (experimental)/propeller thrust model/simulink model/propeller1 ==
  Ω : Inport
  1/2*rho*D^4*kt : Gain  Gain=1/2*rho*D^4*kt
  Abs : Abs
  Product : Product
  T : Outport
  wires:
  Abs/1 -> Product/2
  Ω/1 -> Product/1, Abs/1
  Product/1 -> 1/2*rho*D^4*kt/1  "Ω^2"
  1/2*rho*D^4*kt/1 -> T/1  "T"
